simulink model "SMC_simulacion"  (R2016a)
settings: Solver=ode45  StartTime=0.0  StopTime=10.0  MaxStep=0.02  RelTol=1e-3
libraries: arduino_io_lib x5
settings Model: Creator=Administrador  LastModifiedBy=i95sa
settings DataIOCC: LimitDataPoints=on  SaveFormat=Array  SignalLoggingSaveFormat=ModelDataLogs
settings OptimizationCC: ExpressionDepthLimit=2147483647  InitFltsAndDblsToZero=on
settings DebuggingCC: UnderspecifiedInitializationDetection=Classic  MergeDetectMultiDrivingBlocksExec=none  SolverPrmCheckMsg=warning  FcnCallInpInsideContextMsg=UseLocalSettings  StateNameClashWarn=warning
settings HardwareCC: ProdBitPerPointer=32  ProdLargestAtomicFloat=None  ProdIntDivRoundTo=Undefined  ProdEndianess=Unspecified  ProdWordSize=32  ProdHWDeviceType=32-bit Generic
settings ModelReferenceCC: PropagateSignalLabelsOutOfModel=off
settings GRTTargetCC: CombineOutputUpdateFcns=off  GRTInterface=on
settings ConfigComp: CovModelRefEnable=Off

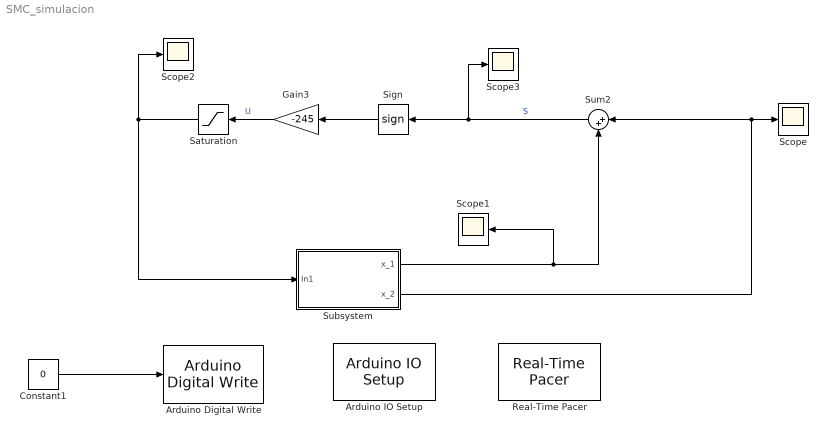
== system SMC_simulacion ==
  Arduino Digital Write : arduino_io_lib/Arduino Digital Write  arduinoVar=Existing workspace arduino variable #1  arduinoPin=6  T=0.1
  Arduino IO Setup : arduino_io_lib/Arduino IO Setup  Priority=3  arduinoVar=Existing workspace arduino variable #1  workspaceVarName=a  comPort=4
  Constant1 : Constant  Value=0
  Gain3 : Gain  Gain=-245
  Real-Time Pacer : arduino_io_lib/Real-Time Pacer  simTimePerRealTime=1
  Saturation : Saturate  UpperLimit=255  LowerLimit=0
  Scope{,1..3} (4 alike) : Scope
  Sign : Signum  ZeroCross=off
  Subsystem : Subsystem
  Sum2 : Sum  Inputs=|++
  wires:
  Sum2/1 -> Scope3/1, Sign/1  "S"
  Sign/1 -> Gain3/1
  Gain3/1 -> Saturation/1  "U"
  Subsystem/1(x_1) -> Sum2/2, Scope1/1
  Subsystem/2(x_2) -> Sum2/1, Scope/1
  Saturation/1 -> Subsystem/1(In1), Scope2/1
  Constant1/1 -> Arduino Digital Write/1

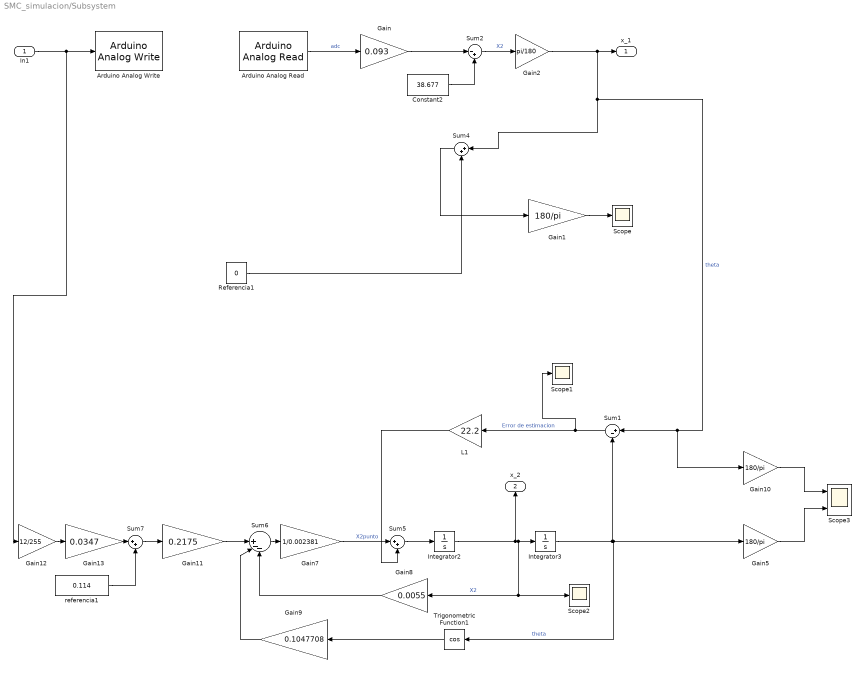
== system SMC_simulacion/Subsystem ==
  In1 : Inport
  Arduino Analog Read : arduino_io_lib/Arduino Analog Read  arduinoVar=Existing workspace arduino variable #1  arduinoPin=0  T=0.1
  Arduino Analog Write : arduino_io_lib/Arduino Analog Write  arduinoVar=Existing workspace arduino variable #1  arduinoPin=7  T=0.1
  Constant2 : Constant  Value=38.677
  Gain : Gain  Gain=0.093
  Gain1 : Gain  Gain=180/pi
  Gain10 : Gain  Gain=180/pi
  Gain11 : Gain  Gain=0.2175
  Gain12 : Gain  Gain=12/255
  Gain13 : Gain  Gain=0.0347
  Gain2 : Gain  Gain=pi/180
  Gain5 : Gain  Gain=180/pi
  Gain7 : Gain  Gain=1/0.002381
  Gain8 : Gain  Gain=0.0055
  Gain9 : Gain  Gain=0.1047708
  Integrator2 : Integrator
  Integrator3 : Integrator  InitialCondition=-0.65
  L1 : Gain  Gain=22.2
  Referencia1 : Constant  Value=0
  Scope : Scope
  Scope1 : Scope
  Scope2 : Scope
  Scope3 : Scope  NumInputPorts=2
  Sum1 : Sum  Inputs=|+-
  Sum2 : Sum  Inputs=|-+
  Sum4 : Sum  Inputs=|++
  Sum5 : Sum  Inputs=|++
  Sum6 : Sum  Inputs=||+--
  Sum7 : Sum  Inputs=|++
  Trigonometric Function1 : Trigonometry  Operator=cos
  referencia1 : Constant  Value=0.114
  x_1 : Outport
  x_2 : Outport  Port=2
  wires:
  In1/1 -> Gain12/1, Arduino Analog Write/1
  Sum4/1 -> Gain1/1
  Referencia1/1 -> Sum4/2
  Gain1/1 -> Scope/1
  Arduino Analog Read/1 -> Gain/1  "adc"
  Gain/1 -> Sum2/1
  Constant2/1 -> Sum2/2
  Sum2/1 -> Gain2/1  "X2"
  Sum6/1 -> Gain7/1
  Trigonometric Function1/1 -> Gain9/1
  Gain8/1 -> Sum6/3
  Gain9/1 -> Sum6/2
  Gain11/1 -> Sum6/1
  referencia1/1 -> Sum7/2
  Sum7/1 -> Gain11/1
  Gain12/1 -> Gain13/1
  Gain13/1 -> Sum7/1
  Gain5/1 -> Scope3/2
  Gain10/1 -> Scope3/1
  Gain2/1 -> Sum1/1, Gain10/1, Sum4/1, x_1/1  "theta"
  Integrator3/1 -> Trigonometric Function1/1, Gain5/1, Sum1/2  "theta"
  Sum1/1 -> Scope1/1, L1/1  "Error de estimacion"
  Integrator2/1 -> Integrator3/1, Scope2/1, Gain8/1, x_2/1  "X2"
  Gain7/1 -> Sum5/1  "X2punto"
  L1/1 -> Sum5/2
  Sum5/1 -> Integrator2/1
